simulink model "sheme"  (R2017b)
settings: Solver=VariableStepAuto  StartTime=0.0  StopTime=600  MaxStep=0.01  RelTol=1e-3
InitFcn:
  | A=[2 8;3 6];
  | b=[2;3];
  | U=ctrb(A,b);
  | rank(U);
  | Ad=[0 1;-256 -32];
  | H=[1 0];
  | U2=obsv(Ad,H);
  | rank(U2);
  | 
  | M=sylv(A,-Ad,b*H);
  | K=H*inv(M);
  | 
  | Af0=[0 1; -0.01 -sqrt(0.02)];
  | bf0=[0;1];
  | syms n11 n12 n21 n22;
  | n=[n11 n12;n21 n22];
  | eqn=n*b==bf0;
  | sol=solve([eqn],[n11, n12, n21, n22]);
  | N=[double(sol.n11) double(sol.n12); double(sol.n21) double(sol.n22)];
  | 
  | Am=A-b*K;
  | Q=eye(2);
  | P=lyap(Am',Q) ;
settings Model: Creator=lida  LastModifiedBy=lida

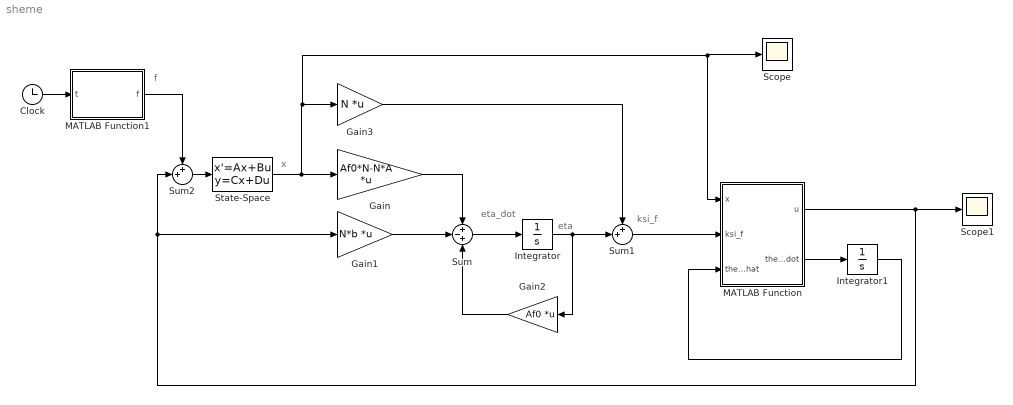
== system sheme ==
  note: ksi_f
  note: eta_dot
  note: eta
  note: f
  note: x
  Clock : Clock
  Gain : Gain  Gain=Af0*N-N*A  Multiplication=Matrix(K*u)
  Gain1 : Gain  Gain=N*b  Multiplication=Matrix(K*u)
  Gain2 : Gain  Gain=Af0  Multiplication=Matrix(K*u)
  Gain3 : Gain  Gain=N  Multiplication=Matrix(K*u)
  Integrator : Integrator
  Integrator1 : Integrator
  MATLAB Function : MATLAB Function  TreatAsAtomicUnit=on
  MATLAB Function1 : MATLAB Function  TreatAsAtomicUnit=on
  Scope : Scope
  Scope1 : Scope
  State-Space : StateSpace  A=A  B=b  C=eye(2)  D=[0;0]  InitialCondition=[1;0]
  Sum : Sum  Inputs=+-+
  Sum1 : Sum  Inputs=++|
  Sum2 : Sum  Inputs=++|
  wires:
  State-Space/1 -> MATLAB Function/1(x), Scope/1, Gain3/1, Gain/1
  Gain/1 -> Sum/1
  Gain1/1 -> Sum/2
  Sum/1 -> Integrator/1
  Integrator/1 -> Sum1/2, Gain2/1
  Gain2/1 -> Sum/3
  Gain3/1 -> Sum1/1
  MATLAB Function/2(theta_dot) -> Integrator1/1
  Integrator1/1 -> MATLAB Function/3(theta_hat)
  Sum1/1 -> MATLAB Function/2(ksi_f)
  Sum2/1 -> State-Space/1
  Clock/1 -> MATLAB Function1/1(t)
  MATLAB Function/1(u) -> Gain1/1, Sum2/2, Scope1/1
  MATLAB Function1/1(f) -> Sum2/1

== matlab function sheme/MATLAB Function1 ==
  data: t input; f output
function f = fcn(t)

f=cos(2*t);

== matlab function sheme/MATLAB Function ==
  data: x input; u output; ksi_f input; theta_hat input; theta_dot output; P parameter; b parameter; K parameter
function [u,theta_dot] = fcn(x,ksi_f,theta_hat, P, b, K)
gamma=100;
u=-K*x-theta_hat'*ksi_f;
theta_dot=gamma*ksi_f*b'*P*x;
